simulink model "testBoom"  (R2021a)
settings: Solver=VariableStepAuto  StartTime=0.0  StopTime=Torb  RelTol=1e-3
settings Model: DataDictionary=databus.sldd  Creator=Laura  LastModifiedBy=Laura

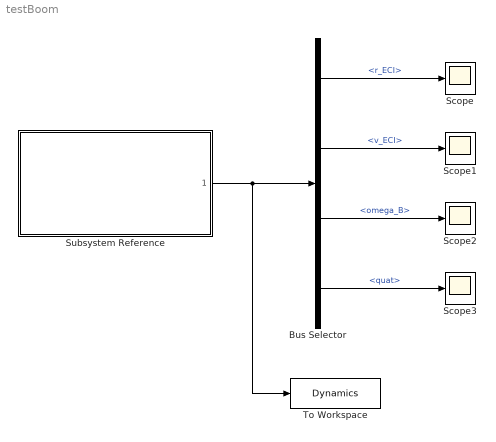
== system testBoom ==
  Bus Selector : BusSelector  OutputSignals=r_ECI,v_ECI,omega_B,quat
  Scope{,1..3} (4 alike) : Scope
  Subsystem Reference : Subsystem  ReferencedSubsystem=SCDynamics_FreeTorque
  To Workspace : ToWorkspace  VariableName=Dynamics  SaveFormat=Timeseries  SampleTime=-1
  wires:
  Subsystem Reference/1 -> To Workspace/1, Bus Selector/1
  Bus Selector/3 -> Scope2/1  "<omega_B>"
  Bus Selector/2 -> Scope1/1  "<v_ECI>"
  Bus Selector/4 -> Scope3/1  "<quat>"
  Bus Selector/1 -> Scope/1  "<r_ECI>"
